simulink model "dsp_blr_hikaku_nakamura_futagi"  (R2018a)
settings: Solver=VariableStepAuto  StartTime=0.0  StopTime=100e-6  RelTol=1e-3
values from neighbouring files (symbols this model uses):
  BASELINE = 0    [dsp_blr.mat]
libraries: xbsIndex_r4 x934, xrbsSSR_Library x35, simulink x3, dspsigattribs x2, hdlsllib x2
(part 1 of 6)
settings Model: Creator=1905p  LastModifiedBy=1905p

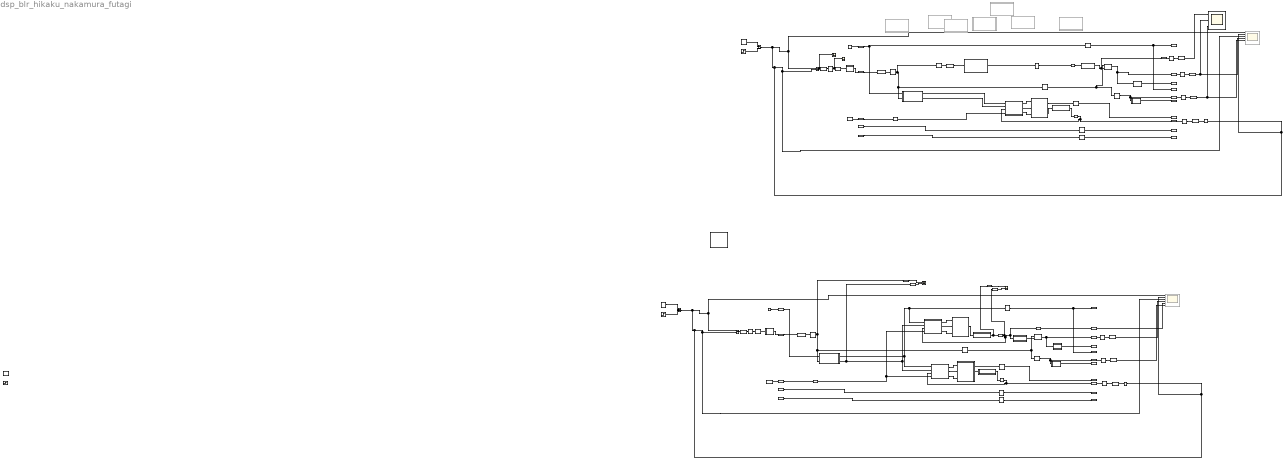
== system dsp_blr_hikaku_nakamura_futagi ==
  note: ここのタイミングはbsp_blr_x.slxのほうで直す
  note: [a:b]を8個用意したが、[0:15]1個ではダメ?
      | 中身は全部同じだった
  note: [a:b]とShiftで入力のvectorと同じ大きさになるようにした
  note: これを入れいるとなぜか上手くいく
  note: 128bitを16bit×8に分け、
      | 足し合わせる
  note: 16×8=128bit
      | のスカラー
  note: 16bit
      | ...
      | 16bit
      | ↑
      | 8行のベクトル
  note: DAC controller
  note: digital_baseline_correction
  note: DSP_module
  note: DAC controller
  note: DSP_module
  note: 16×8=128bit
      | のスカラー
  note: 16bit
      | ...
      | 16bit
      | ↑
      | 8行のベクトル
  note: ここのタイミングはbsp_blr_x.slxのほうで直す
  " System Generator" : xbsIndex_r4/ System Generator  Tag=genX  xilinxfamily=zynquplusRFSOC  part=xczu29dr  speed=-1-e  package=ffvf1760  synthesis_tool=Vivado  clock_wrapper=Clock Enables  directory=C:/Users/1905p/git_repos/KRD/ip_repos/SysGen_outputs/dsp_blr  proj_type=Vivado  Synth_file=Vivado Synthesis Defaults  Impl_file=Vivado Implementation Defaults  testbench=on  simulink_period=8e-9  sysclk_period=8  dcm_input_clock_period=10  incr_netlist=off  trim_vbits=Everywhere in SubSystem  dbl_ovrd=According to Block Masks  core_generation=According to Block Masks  run_coregen=off  deprecated_control=off  eval_field=0  block_type=sysgen
  +cut : Subsystem
  8sample_average 1 : Subsystem
  8sample_average 3 : Subsystem
  "?1" : xbsIndex_r4/Convert  gui_display_data_type=Fixed-point  arith_type="Signed  (2's comp)"  n_bits=16  bin_pt=4  float_type=Single  exp_bits=8  fraction_bits=24  quantization=Truncate  overflow=Saturate  en=off  latency=1  pipeline=off  dbl_ovrd=off  block_type=convert
  Ave10 : Subsystem  Commented=on
  Ave11 : Subsystem
  Ave12 : Subsystem  Commented=on
  Ave5 : Subsystem  Commented=on
  Ave6 : Subsystem  Commented=on
  Ave7 : Subsystem  Commented=on
  Ave8 : Subsystem  Commented=on
  Ave9 : Subsystem  Commented=on
  Buffer1 : Buffer  N=8  OutputFrames=off
  Buffer6 : Buffer  N=8  OutputFrames=off
  Convert 2-D to 1-D1 : dspsigattribs/Convert 2-D to 1-D
      settings: SourceProductName=DSP System Toolbox  SourceProductBaseCode=DS
  Convert 2-D to 1-D6 : dspsigattribs/Convert 2-D to 1-D
      settings: SourceProductName=DSP System Toolbox  SourceProductBaseCode=DS
  Convert1 : xbsIndex_r4/Convert  gui_display_data_type=Fixed-point  arith_type="Signed  (2's comp)"  n_bits=16  bin_pt=4  float_type=Single  exp_bits=8  fraction_bits=24  quantization=Truncate  overflow=Wrap  en=off  latency=0  pipeline=off  dbl_ovrd=off  block_type=convert
  Convert2 : xbsIndex_r4/Convert  gui_display_data_type=Fixed-point  arith_type="Signed  (2's comp)"  n_bits=16  bin_pt=4  float_type=Single  exp_bits=8  fraction_bits=24  quantization=Truncate  overflow=Wrap  en=off  latency=0  pipeline=off  dbl_ovrd=off  block_type=convert
  DAC_M_AXIS_TDATA1 : xbsIndex_r4/Gateway Out  inherit_from_input=on  hdl_port=on  rows=1  columns=1  UseAsDAC=off  DACChannel='1'  interface=None  automatic_assignment=on  address_offset=hex2dec('00')  intf_name=''  intf_description=''  timing_constraint=None  locs_specified=off  LOCs={}  io_standard={}  block_type=gatewayout
  DAC_M_AXIS_TDATA2 : xbsIndex_r4/Gateway Out  inherit_from_input=on  hdl_port=on  rows=1  columns=1  UseAsDAC=off  DACChannel='1'  interface=None  automatic_assignment=on  address_offset=hex2dec('00')  intf_name=''  intf_description=''  timing_constraint=None  locs_specified=off  LOCs={}  io_standard={}  block_type=gatewayout
  DAC_M_AXIS_TVALID1 : xbsIndex_r4/Gateway Out  inherit_from_input=off  hdl_port=on  rows=1  columns=1  UseAsDAC=off  DACChannel='1'  interface=None  automatic_assignment=on  address_offset=hex2dec('00')  intf_name=''  intf_description=''  timing_constraint=None  locs_specified=off  LOCs={}  io_standard={}  block_type=gatewayout
  DAC_M_AXIS_TVALID2 : xbsIndex_r4/Gateway Out  inherit_from_input=off  hdl_port=on  rows=1  columns=1  UseAsDAC=off  DACChannel='1'  interface=None  automatic_assignment=on  address_offset=hex2dec('00')  intf_name=''  intf_description=''  timing_constraint=None  locs_specified=off  LOCs={}  io_standard={}  block_type=gatewayout
  DBL_Scalar2Vector1 : Subsystem
  DBL_Scalar2Vector2 : Subsystem
  DIGITAL_BASELINE4 : xbsIndex_r4/Gateway Out  inherit_from_input=on  hdl_port=on  rows=1  columns=1  UseAsDAC=off  DACChannel='1'  interface=None  automatic_assignment=on  address_offset=hex2dec('00')  intf_name=''  intf_description=''  timing_constraint=None  locs_specified=off  LOCs={}  io_standard={}  block_type=gatewayout
  DSP_M_AXIS_TDATA1 : xbsIndex_r4/Gateway Out  inherit_from_input=on  hdl_port=on  rows=1  columns=1  UseAsDAC=off  DACChannel='1'  interface=None  automatic_assignment=on  address_offset=hex2dec('00')  intf_name=''  intf_description=''  timing_constraint=None  locs_specified=off  LOCs={}  io_standard={}  block_type=gatewayout
  DSP_M_AXIS_TDATA6 : xbsIndex_r4/Gateway Out  inherit_from_input=on  hdl_port=on  rows=1  columns=1  UseAsDAC=off  DACChannel='1'  interface=None  automatic_assignment=on  address_offset=hex2dec('00')  intf_name=''  intf_description=''  timing_constraint=None  locs_specified=off  LOCs={}  io_standard={}  block_type=gatewayout
  DSP_M_AXIS_TDATA_debug1 : xrbsSSR_Library/Vector Real Gateway Out  inherit_from_input=on  hdl_port=off  rows=1  columns=1  UseAsDAC=off  DACChannel='1'  interface=None  automatic_assignment=on  address_offset=hex2dec('00')  intf_name=''  intf_description=''  timing_constraint=None  locs_specified=off  LOCs={}  io_standard={}  block_type=realgatewayout_ssr  sg_ssr=8  sg_ssr_prev=8  sg_ssr_name=vect_real_gwayout
      settings: SourceProductName=Xilinx SSR Blockset  infoedit=The Vector Real Gateway out block converts Xilinx fixed-point or floating-point type vector inputs into vector ouputs of type Simulink integer, single, double, or fixed-point.<br><br>Hardware notes: In hardware these blocks become top level output ports or are discarded, depending on how they are configured.
  DSP_M_AXIS_TDATA_debug2 : xrbsSSR_Library/Vector Real Gateway Out  inherit_from_input=on  hdl_port=off  rows=1  columns=1  UseAsDAC=off  DACChannel='1'  interface=None  automatic_assignment=on  address_offset=hex2dec('00')  intf_name=''  intf_description=''  timing_constraint=None  locs_specified=off  LOCs={}  io_standard={}  block_type=realgatewayout_ssr  sg_ssr=8  sg_ssr_prev=8  sg_ssr_name=vect_real_gwayout
      settings: SourceProductName=Xilinx SSR Blockset  infoedit=The Vector Real Gateway out block converts Xilinx fixed-point or floating-point type vector inputs into vector ouputs of type Simulink integer, single, double, or fixed-point.<br><br>Hardware notes: In hardware these blocks become top level output ports or are discarded, depending on how they are configured.
  DSP_M_AXIS_TDATA_debug7 : xrbsSSR_Library/Vector Real Gateway Out  inherit_from_input=on  hdl_port=off  rows=1  columns=1  UseAsDAC=off  DACChannel='1'  interface=None  automatic_assignment=on  address_offset=hex2dec('00')  intf_name=''  intf_description=''  timing_constraint=None  locs_specified=off  LOCs={}  io_standard={}  block_type=realgatewayout_ssr  sg_ssr=8  sg_ssr_prev=8  sg_ssr_name=vect_real_gwayout
      settings: SourceProductName=Xilinx SSR Blockset  infoedit=The Vector Real Gateway out block converts Xilinx fixed-point or floating-point type vector inputs into vector ouputs of type Simulink integer, single, double, or fixed-point.<br><br>Hardware notes: In hardware these blocks become top level output ports or are discarded, depending on how they are configured.
  DSP_M_AXIS_TVALID1 : xbsIndex_r4/Gateway Out  inherit_from_input=on  hdl_port=on  rows=1  columns=1  UseAsDAC=off  DACChannel='1'  interface=None  automatic_assignment=on  address_offset=hex2dec('00')  intf_name=''  intf_description=''  timing_constraint=None  locs_specified=off  LOCs={}  io_standard={}  block_type=gatewayout
  DSP_M_AXIS_TVALID6 : xbsIndex_r4/Gateway Out  inherit_from_input=on  hdl_port=on  rows=1  columns=1  UseAsDAC=off  DACChannel='1'  interface=None  automatic_assignment=on  address_offset=hex2dec('00')  intf_name=''  intf_description=''  timing_constraint=None  locs_specified=off  LOCs={}  io_standard={}  block_type=gatewayout
  DSP_Vector2Scalar1 : Subsystem
  DSP_Vector2Scalar6 : Subsystem
  DSP_delay1 : xrbsSSR_Library/Vector Delay  sg_latency=7  infoeditControl=Selection of Reset will increase slice count due to use of real FFs and instead of SRLs  en=off  vectorize_en=off  rst=off  reg_retiming=off  block_type=delay_ssr  dbl_ovrd=off  sg_ssr=8  sg_ssr_prev=8  sg_ssr_name=vect_delay
      settings: SourceProductName=Xilinx SSR Blockset
  DSP_delay6 : xrbsSSR_Library/Vector Delay  sg_latency=6  infoeditControl=Selection of Reset will increase slice count due to use of real FFs and instead of SRLs  en=off  vectorize_en=off  rst=off  reg_retiming=off  block_type=delay_ssr  dbl_ovrd=off  sg_ssr=8  sg_ssr_prev=8  sg_ssr_name=vect_delay
      settings: SourceProductName=Xilinx SSR Blockset
  Delay1 : xbsIndex_r4/Delay  rst=off  infoeditControl=Selection of Reset will increase slice count due to use of real FFs and instead of SRLs  en=off  latency=6  reg_retiming=off  dbl_ovrd=off  block_type=delay
  Delay6 : xbsIndex_r4/Delay  rst=off  infoeditControl=Selection of Reset will increase slice count due to use of real FFs and instead of SRLs  en=off  latency=6  reg_retiming=off  dbl_ovrd=off  block_type=delay
  Gateway Out2 : xbsIndex_r4/Gateway Out  inherit_from_input=off  hdl_port=on  rows=1  columns=1  UseAsDAC=off  DACChannel='1'  interface=None  automatic_assignment=on  address_offset=hex2dec('00')  intf_name=''  intf_description=''  timing_constraint=None  locs_specified=off  LOCs={}  io_standard={}  block_type=gatewayout
  Gateway Out3 : xbsIndex_r4/Gateway Out  inherit_from_input=off  hdl_port=on  rows=1  columns=1  UseAsDAC=off  DACChannel='1'  interface=None  automatic_assignment=on  address_offset=hex2dec('00')  intf_name=''  intf_description=''  timing_constraint=None  locs_specified=off  LOCs={}  io_standard={}  block_type=gatewayout
  Gateway Out6 : xbsIndex_r4/Gateway Out  inherit_from_input=off  hdl_port=on  rows=1  columns=1  UseAsDAC=off  DACChannel='1'  interface=None  automatic_assignment=on  address_offset=hex2dec('00')  intf_name=''  intf_description=''  timing_constraint=None  locs_specified=off  LOCs={}  io_standard={}  block_type=gatewayout
  HGAIN_Vector2Scalar1 : Subsystem
  HGAIN_Vector2Scalar6 : Subsystem
  HGAIN_delay1 : xrbsSSR_Library/Vector Delay  sg_latency=1  infoeditControl=Selection of Reset will increase slice count due to use of real FFs and instead of SRLs  en=off  vectorize_en=off  rst=off  reg_retiming=off  block_type=delay_ssr  dbl_ovrd=off  sg_ssr=8  sg_ssr_prev=8  sg_ssr_name=vect_delay
      settings: SourceProductName=Xilinx SSR Blockset
  HGAIN_delay6 : xrbsSSR_Library/Vector Delay  sg_latency=1  infoeditControl=Selection of Reset will increase slice count due to use of real FFs and instead of SRLs  en=off  vectorize_en=off  rst=off  reg_retiming=off  block_type=delay_ssr  dbl_ovrd=off  sg_ssr=8  sg_ssr_prev=8  sg_ssr_name=vect_delay
      settings: SourceProductName=Xilinx SSR Blockset
  H_GAIN_BASELINE1 : xbsIndex_r4/Gateway In  gui_display_data_type=Fixed-point  arith_type="Signed  (2's comp)"  n_bits=13  bin_pt=0  preci_type=Single  exp_width=8  frac_width=24  rows=1  columns=1  quantization=Truncate  overflow=Wrap  period=8e-9  UseAsADC=off  ADCChannel='1'  interface=None  automatic_assignment=on  address_offset=hex2dec('00')  intf_name=''  intf_description=''  default_value=0  timing_constraint=None  locs_specified=off  LOCs={}  io_standard={}  inherit_from_input=off  hdl_port=on  dbl_ovrd=off  block_type=gatewayin
  H_GAIN_BASELINE2 : xbsIndex_r4/Gateway In  gui_display_data_type=Fixed-point  arith_type="Signed  (2's comp)"  n_bits=13  bin_pt=0  preci_type=Single  exp_width=8  frac_width=24  rows=1  columns=1  quantization=Truncate  overflow=Wrap  period=8e-9  UseAsADC=off  ADCChannel='1'  interface=None  automatic_assignment=on  address_offset=hex2dec('00')  intf_name=''  intf_description=''  default_value=0  timing_constraint=None  locs_specified=off  LOCs={}  io_standard={}  inherit_from_input=off  hdl_port=on  dbl_ovrd=off  block_type=gatewayin
  H_M_AXIS_TDATA1 : xbsIndex_r4/Gateway Out  inherit_from_input=on  hdl_port=on  rows=1  columns=1  UseAsDAC=off  DACChannel='1'  interface=None  automatic_assignment=on  address_offset=hex2dec('00')  intf_name=''  intf_description=''  timing_constraint=None  locs_specified=off  LOCs={}  io_standard={}  block_type=gatewayout
  H_M_AXIS_TDATA6 : xbsIndex_r4/Gateway Out  inherit_from_input=on  hdl_port=on  rows=1  columns=1  UseAsDAC=off  DACChannel='1'  interface=None  automatic_assignment=on  address_offset=hex2dec('00')  intf_name=''  intf_description=''  timing_constraint=None  locs_specified=off  LOCs={}  io_standard={}  block_type=gatewayout
  H_M_AXIS_TDATA_debug1 : xrbsSSR_Library/Vector Real Gateway Out  inherit_from_input=on  hdl_port=off  rows=1  columns=1  UseAsDAC=off  DACChannel='1'  interface=None  automatic_assignment=on  address_offset=hex2dec('00')  intf_name=''  intf_description=''  timing_constraint=None  locs_specified=off  LOCs={}  io_standard={}  block_type=realgatewayout_ssr  sg_ssr=8  sg_ssr_prev=8  sg_ssr_name=vect_real_gwayout
      settings: SourceProductName=Xilinx SSR Blockset  infoedit=The Vector Real Gateway out block converts Xilinx fixed-point or floating-point type vector inputs into vector ouputs of type Simulink integer, single, double, or fixed-point.<br><br>Hardware notes: In hardware these blocks become top level output ports or are discarded, depending on how they are configured.
  H_M_AXIS_TDATA_debug6 : xrbsSSR_Library/Vector Real Gateway Out  inherit_from_input=on  hdl_port=off  rows=1  columns=1  UseAsDAC=off  DACChannel='1'  interface=None  automatic_assignment=on  address_offset=hex2dec('00')  intf_name=''  intf_description=''  timing_constraint=None  locs_specified=off  LOCs={}  io_standard={}  block_type=realgatewayout_ssr  sg_ssr=8  sg_ssr_prev=8  sg_ssr_name=vect_real_gwayout
      settings: SourceProductName=Xilinx SSR Blockset  infoedit=The Vector Real Gateway out block converts Xilinx fixed-point or floating-point type vector inputs into vector ouputs of type Simulink integer, single, double, or fixed-point.<br><br>Hardware notes: In hardware these blocks become top level output ports or are discarded, depending on how they are configured.
  H_M_AXIS_TVALID1 : xbsIndex_r4/Gateway Out  inherit_from_input=on  hdl_port=on  rows=1  columns=1  UseAsDAC=off  DACChannel='1'  interface=None  automatic_assignment=on  address_offset=hex2dec('00')  intf_name=''  intf_description=''  timing_constraint=None  locs_specified=off  LOCs={}  io_standard={}  block_type=gatewayout
  H_M_AXIS_TVALID6 : xbsIndex_r4/Gateway Out  inherit_from_input=on  hdl_port=on  rows=1  columns=1  UseAsDAC=off  DACChannel='1'  interface=None  automatic_assignment=on  address_offset=hex2dec('00')  intf_name=''  intf_description=''  timing_constraint=None  locs_specified=off  LOCs={}  io_standard={}  block_type=gatewayout
  H_S_AXIS_TDATA1 : xbsIndex_r4/Gateway In  gui_display_data_type=Fixed-point  arith_type=Unsigned  n_bits=128  bin_pt=0  preci_type=Single  exp_width=8  frac_width=24  rows=1  columns=1  quantization=Truncate  overflow=Wrap  period=8e-9  UseAsADC=off  ADCChannel='1'  interface=None  automatic_assignment=on  address_offset=hex2dec('00')  intf_name=''  intf_description=''  default_value=0  timing_constraint=None  locs_specified=off  LOCs={}  io_standard={}  inherit_from_input=off  hdl_port=on  dbl_ovrd=off  block_type=gatewayin
  H_S_AXIS_TDATA6 : xbsIndex_r4/Gateway In  gui_display_data_type=Fixed-point  arith_type=Unsigned  n_bits=128  bin_pt=0  preci_type=Single  exp_width=8  frac_width=24  rows=1  columns=1  quantization=Truncate  overflow=Wrap  period=8e-9  UseAsADC=off  ADCChannel='1'  interface=None  automatic_assignment=on  address_offset=hex2dec('00')  intf_name=''  intf_description=''  default_value=0  timing_constraint=None  locs_specified=off  LOCs={}  io_standard={}  inherit_from_input=off  hdl_port=on  dbl_ovrd=off  block_type=gatewayin
  H_S_AXIS_TVALID1 : xbsIndex_r4/Gateway In  gui_display_data_type=Boolean  arith_type=Boolean  n_bits=16  bin_pt=14  preci_type=Single  exp_width=8  frac_width=24  rows=1  columns=1  quantization="Round  (unbiased: +/- Inf)"  overflow=Saturate  period=8e-9  UseAsADC=off  ADCChannel='1'  interface=None  automatic_assignment=on  address_offset=hex2dec('00')  intf_name=''  intf_description=''  default_value=0  timing_constraint=None  locs_specified=off  LOCs={}  io_standard={}  inherit_from_input=off  hdl_port=on  dbl_ovrd=off  block_type=gatewayin
  H_S_AXIS_TVALID6 : xbsIndex_r4/Gateway In  gui_display_data_type=Boolean  arith_type=Boolean  n_bits=16  bin_pt=14  preci_type=Single  exp_width=8  frac_width=24  rows=1  columns=1  quantization="Round  (unbiased: +/- Inf)"  overflow=Saturate  period=8e-9  UseAsADC=off  ADCChannel='1'  interface=None  automatic_assignment=on  address_offset=hex2dec('00')  intf_name=''  intf_description=''  default_value=0  timing_constraint=None  locs_specified=off  LOCs={}  io_standard={}  inherit_from_input=off  hdl_port=on  dbl_ovrd=off  block_type=gatewayin
  L_GAIN_TDATA_delay1 : xbsIndex_r4/Delay  rst=off  infoeditControl=Selection of Reset will increase slice count due to use of real FFs and instead of SRLs  en=off  latency=6  reg_retiming=off  dbl_ovrd=off  block_type=delay
  L_GAIN_TDATA_delay6 : xbsIndex_r4/Delay  rst=off  infoeditControl=Selection of Reset will increase slice count due to use of real FFs and instead of SRLs  en=off  latency=6  reg_retiming=off  dbl_ovrd=off  block_type=delay
  L_GAIN_TVALID_delay1 : xbsIndex_r4/Delay  rst=off  infoeditControl=Selection of Reset will increase slice count due to use of real FFs and instead of SRLs  en=off  latency=6  reg_retiming=off  dbl_ovrd=off  block_type=delay
  L_GAIN_TVALID_delay6 : xbsIndex_r4/Delay  rst=off  infoeditControl=Selection of Reset will increase slice count due to use of real FFs and instead of SRLs  en=off  latency=6  reg_retiming=off  dbl_ovrd=off  block_type=delay
  L_M_AXIS_TDATA1 : xbsIndex_r4/Gateway Out  inherit_from_input=on  hdl_port=on  rows=1  columns=1  UseAsDAC=off  DACChannel='1'  interface=None  automatic_assignment=on  address_offset=hex2dec('00')  intf_name=''  intf_description=''  timing_constraint=None  locs_specified=off  LOCs={}  io_standard={}  block_type=gatewayout
  L_M_AXIS_TDATA6 : xbsIndex_r4/Gateway Out  inherit_from_input=on  hdl_port=on  rows=1  columns=1  UseAsDAC=off  DACChannel='1'  interface=None  automatic_assignment=on  address_offset=hex2dec('00')  intf_name=''  intf_description=''  timing_constraint=None  locs_specified=off  LOCs={}  io_standard={}  block_type=gatewayout
  L_M_AXIS_TVALID1 : xbsIndex_r4/Gateway Out  inherit_from_input=on  hdl_port=on  rows=1  columns=1  UseAsDAC=off  DACChannel='1'  interface=None  automatic_assignment=on  address_offset=hex2dec('00')  intf_name=''  intf_description=''  timing_constraint=None  locs_specified=off  LOCs={}  io_standard={}  block_type=gatewayout
  L_M_AXIS_TVALID6 : xbsIndex_r4/Gateway Out  inherit_from_input=on  hdl_port=on  rows=1  columns=1  UseAsDAC=off  DACChannel='1'  interface=None  automatic_assignment=on  address_offset=hex2dec('00')  intf_name=''  intf_description=''  timing_constraint=None  locs_specified=off  LOCs={}  io_standard={}  block_type=gatewayout
  L_S_AXIS_TDATA1 : xbsIndex_r4/Gateway In  gui_display_data_type=Fixed-point  arith_type=Unsigned  n_bits=32  bin_pt=0  preci_type=Single  exp_width=8  frac_width=24  rows=1  columns=1  quantization=Truncate  overflow=Wrap  period=8e-9  UseAsADC=off  ADCChannel='1'  interface=None  automatic_assignment=on  address_offset=hex2dec('00')  intf_name=''  intf_description=''  default_value=0  timing_constraint=None  locs_specified=off  LOCs={}  io_standard={}  inherit_from_input=off  hdl_port=on  dbl_ovrd=off  block_type=gatewayin
  L_S_AXIS_TDATA6 : xbsIndex_r4/Gateway In  gui_display_data_type=Fixed-point  arith_type=Unsigned  n_bits=32  bin_pt=0  preci_type=Single  exp_width=8  frac_width=24  rows=1  columns=1  quantization=Truncate  overflow=Wrap  period=8e-9  UseAsADC=off  ADCChannel='1'  interface=None  automatic_assignment=on  address_offset=hex2dec('00')  intf_name=''  intf_description=''  default_value=0  timing_constraint=None  locs_specified=off  LOCs={}  io_standard={}  inherit_from_input=off  hdl_port=on  dbl_ovrd=off  block_type=gatewayin
  L_S_AXIS_TVALID1 : xbsIndex_r4/Gateway In  gui_display_data_type=Boolean  arith_type=Boolean  n_bits=16  bin_pt=14  preci_type=Single  exp_width=8  frac_width=24  rows=1  columns=1  quantization="Round  (unbiased: +/- Inf)"  overflow=Saturate  period=8e-9  UseAsADC=off  ADCChannel='1'  interface=None  automatic_assignment=on  address_offset=hex2dec('00')  intf_name=''  intf_description=''  default_value=0  timing_constraint=None  locs_specified=off  LOCs={}  io_standard={}  inherit_from_input=off  hdl_port=on  dbl_ovrd=off  block_type=gatewayin
  L_S_AXIS_TVALID6 : xbsIndex_r4/Gateway In  gui_display_data_type=Boolean  arith_type=Boolean  n_bits=16  bin_pt=14  preci_type=Single  exp_width=8  frac_width=24  rows=1  columns=1  quantization="Round  (unbiased: +/- Inf)"  overflow=Saturate  period=8e-9  UseAsADC=off  ADCChannel='1'  interface=None  automatic_assignment=on  address_offset=hex2dec('00')  intf_name=''  intf_description=''  default_value=0  timing_constraint=None  locs_specified=off  LOCs={}  io_standard={}  inherit_from_input=off  hdl_port=on  dbl_ovrd=off  block_type=gatewayin
  Output data Type Conversion DSP1 : DataTypeConversion  OutDataTypeStr=double
  Output data Type Conversion DSP2 : DataTypeConversion  OutDataTypeStr=double
  Output data Type Conversion DSP7 : DataTypeConversion  OutDataTypeStr=double
  Output data Type Conversion HGAIN1 : DataTypeConversion  OutDataTypeStr=double
  Output data Type Conversion HGAIN6 : DataTypeConversion  OutDataTypeStr=double
  Output data Type Conversion1 : DataTypeConversion  OutDataTypeStr=double
  Output data Type Conversion2 : DataTypeConversion  OutDataTypeStr=double
  Scalar2Vector1 : xrbsSSR_Library/Scalar2Vector  Width=16  sg_ssr=8  sg_ssr_prev=8  sg_ssr_name=vect_Scalar2Vector  block_type=scalar2vector_ssr
      settings: SourceProductName=Xilinx SSR Blockset
  Scalar2Vector6 : xrbsSSR_Library/Scalar2Vector  Width=16  sg_ssr=8  sg_ssr_prev=8  sg_ssr_name=vect_Scalar2Vector  block_type=scalar2vector_ssr
      settings: SourceProductName=Xilinx SSR Blockset
  Scope : Scope  NumInputPorts=3
  Scope4 : Scope  NumInputPorts=2
  Scope6 : Scope
  Scope7 : Scope
  Scope8 : Scope  NumInputPorts=2
  Scope_xil1 : Scope  Commented=on  NumInputPorts=6
  Scope_xil2 : Scope  Commented=on  NumInputPorts=6
  Src Switch1 : ManualSwitch
  Src Switch2 : ManualSwitch  CurrentSetting=0
  Src data Type Conversion1 : DataTypeConversion  OutMin=-2048  OutMax=2047  OutDataTypeStr=fixdt(1,16,4)
  Src data Type Conversion6 : DataTypeConversion  OutMin=-2048  OutMax=2047  OutDataTypeStr=fixdt(1,16,4)
  Step1 : Step  Time=50e-6  After=-1024  SampleTime=1e-9
  Step2 : Step  Time=50e-6  After=-1024  SampleTime=1e-9
  Step3 : Step  Time=50e-6  After=-1024  SampleTime=1e-9
  Sum : Sum  Inputs=|+-
  Sum1 : Sum  Inputs=|+-
  Unbuffer DSP1 : Unbuffer
  Unbuffer DSP2 : Unbuffer
  Unbuffer DSP7 : Unbuffer
  Unbuffer HGAIN1 : Unbuffer
  Unbuffer HGAIN6 : Unbuffer
  Unbuffer1 : Unbuffer
  Unbuffer2 : Unbuffer
  Vector AddSub Fabric1 : xrbsSSR_Library/Vector AddSub Fabric  mode=Subtraction  use_carryin=off  use_carryout=off  en=off  sg_latency=1  precision=User Defined  arith_type="Signed  (2's comp)"  n_bits=16  bin_pt=0  quantization=Truncate  overflow=Wrap  use_behavioral_HDL=off  hw_selection=Fabric  pipelined=off  dbl_ovrd=off  block_type=addsub_ssr  sg_ssr=8  sg_ssr_prev=8  sg_ssr_name=vect_addsubfab
      settings: SourceProductName=Xilinx SSR Blockset
  Vector AddSub Fabric2 : xrbsSSR_Library/Vector AddSub Fabric  mode=Subtraction  use_carryin=off  use_carryout=off  en=off  sg_latency=1  precision=User Defined  arith_type="Signed  (2's comp)"  n_bits=16  bin_pt=0  quantization=Truncate  overflow=Wrap  use_behavioral_HDL=off  hw_selection=Fabric  pipelined=off  dbl_ovrd=off  block_type=addsub_ssr  sg_ssr=8  sg_ssr_prev=8  sg_ssr_name=vect_addsubfab
      settings: SourceProductName=Xilinx SSR Blockset
  Vector Real Gateway Out1 : xrbsSSR_Library/Vector Real Gateway Out  inherit_from_input=off  hdl_port=on  rows=1  columns=1  UseAsDAC=off  DACChannel='1'  interface=None  automatic_assignment=on  address_offset=hex2dec('00')  intf_name=''  intf_description=''  timing_constraint=None  locs_specified=off  LOCs={}  io_standard={}  block_type=realgatewayout_ssr  sg_ssr=8  sg_ssr_prev=8  sg_ssr_name=vect_real_gwayout
      settings: SourceProductName=Xilinx SSR Blockset  infoedit=The Vector Real Gateway out block converts Xilinx fixed-point or floating-point type vector inputs into vector ouputs of type Simulink integer, single, double, or fixed-point.<br><br>Hardware notes: In hardware these blocks become top level output ports or are discarded, depending on how they are configured.
  Vector Reinterpret : xrbsSSR_Library/Vector Reinterpret  sg_ssr=8  sg_ssr_prev=8  force_arith_type=on  arith_type=Unsigned  force_bin_pt=on  bin_pt=0  block_type=reinterpret_ssr
      settings: SourceProductName=Xilinx SSR Blockset  infoedit="The Vector Reinterpret block Changes vector input signal type without altering the binary representation. You can change the signal between signed and unsigned, and relocate the binary point.<br><br>Hardware notes: In hardware this block costs nothing.<br><br>Example:  Suppose the input is 6 bits wide, signed, with 2 fractional bits, and the output is forced to unsigned with 0 fractional bits.  Then an input of -2.0 (1110.00 in binary 2's complement) becomes an output of 56 (111000 in binary)."
  Vector Reinterpret1 : xrbsSSR_Library/Vector Reinterpret  sg_ssr=8  sg_ssr_prev=8  force_arith_type=on  arith_type="Signed  (2's comp)"  force_bin_pt=on  bin_pt=4  block_type=reinterpret_ssr
      settings: SourceProductName=Xilinx SSR Blockset  infoedit="The Vector Reinterpret block Changes vector input signal type without altering the binary representation. You can change the signal between signed and unsigned, and relocate the binary point.<br><br>Hardware notes: In hardware this block costs nothing.<br><br>Example:  Suppose the input is 6 bits wide, signed, with 2 fractional bits, and the output is forced to unsigned with 0 fractional bits.  Then an input of -2.0 (1110.00 in binary 2's complement) becomes an output of 56 (111000 in binary)."
  Vector Reinterpret6 : xrbsSSR_Library/Vector Reinterpret  sg_ssr=8  sg_ssr_prev=8  force_arith_type=on  arith_type="Signed  (2's comp)"  force_bin_pt=on  bin_pt=4  block_type=reinterpret_ssr
      settings: SourceProductName=Xilinx SSR Blockset  infoedit="The Vector Reinterpret block Changes vector input signal type without altering the binary representation. You can change the signal between signed and unsigned, and relocate the binary point.<br><br>Hardware notes: In hardware this block costs nothing.<br><br>Example:  Suppose the input is 6 bits wide, signed, with 2 fractional bits, and the output is forced to unsigned with 0 fractional bits.  Then an input of -2.0 (1110.00 in binary 2's complement) becomes an output of 56 (111000 in binary)."
  Vector2Bus1 : Subsystem
  Vector2Bus6 : Subsystem
  Vector2Scalar : xrbsSSR_Library/Vector2Scalar  sg_ssr=8  sg_ssr_prev=8  sg_ssr_name=vect_Vector2Scalar  block_type=vector2scalar_ssr
      settings: SourceProductName=Xilinx SSR Blockset
  Waveform Generator1 : simulink/Sources/Waveform Generator  OutMin=[]  OutMax=[]  OutDataTypeStr=double  SelectedSignal=1  Signals=sin('Amplitude',1024,'Frequency',1000e3,'Phase',0)+square('Amplitude',400,'Frequency',20e6,'Phase',0,'DutyCycle',20)#pulse('Amplitude',1024,'TriggerTime',50e-9,'Duration',50e-9)+step('StepTime',100e-9,'InitialValue',0,'FinalValue',-512)  BlockNames=MultiportSwitch_2ee4ca9575f04b1#MultiportSwitch_74e4ddee714d4bc  SampleTime=1e-9
      settings: SourceProductName=Simulink
  Waveform Generator2 : simulink/Sources/Waveform Generator  OutMin=[]  OutMax=[]  OutDataTypeStr=double  SelectedSignal=1  Signals=sin('Amplitude',1024,'Frequency',1000e3,'Phase',0)+square('Amplitude',400,'Frequency',20e6,'Phase',0,'DutyCycle',20)#pulse('Amplitude',1024,'TriggerTime',50e-9,'Duration',50e-9)+step('StepTime',100e-9,'InitialValue',0,'FinalValue',-512)  BlockNames=MultiportSwitch_2ee4ca9575f04b1#MultiportSwitch_74e4ddee714d4bc  SampleTime=1e-9
      settings: SourceProductName=Simulink
  Waveform Generator3 : simulink/Sources/Waveform Generator  OutMin=[]  OutMax=[]  OutDataTypeStr=double  SelectedSignal=1  Signals=sin('Amplitude',1024,'Frequency',1000e3,'Phase',0)+square('Amplitude',400,'Frequency',20e6,'Phase',0,'DutyCycle',20)#pulse('Amplitude',1024,'TriggerTime',50e-9,'Duration',50e-9)+step('StepTime',100e-9,'InitialValue',0,'FinalValue',-512)  BlockNames=MultiportSwitch_2ee4ca9575f04b1#MultiportSwitch_74e4ddee714d4bc  SampleTime=1e-9
      settings: SourceProductName=Simulink
  baseline1 : Constant  Value=BASELINE  VectorParams1D=off  OutDataTypeStr=Inherit: Inherit via back propagation  SampleTime=1/125e6
  baseline2 : Constant  Value=BASELINE  VectorParams1D=off  OutDataTypeStr=Inherit: Inherit via back propagation  SampleTime=1/125e6
  blr_switch1 : ManualSwitch  CurrentSetting=0
  blr_switch2 : ManualSwitch  CurrentSetting=0
  cast_DBL_out : xbsIndex_r4/Convert  gui_display_data_type=Fixed-point  arith_type="Signed  (2's comp)"  n_bits=16  bin_pt=0  float_type=Single  exp_bits=8  fraction_bits=24  quantization=Truncate  overflow=Wrap  en=off  latency=1  pipeline=off  dbl_ovrd=off  block_type=convert
  convert_to_dac_data2 : xbsIndex_r4/Convert  gui_display_data_type=Fixed-point  arith_type="Signed  (2's comp)"  n_bits=16  bin_pt=4  float_type=Single  exp_bits=8  fraction_bits=24  quantization=Truncate  overflow=Saturate  en=off  latency=1  pipeline=off  dbl_ovrd=off  block_type=convert
  convert_to_dac_input1 : xbsIndex_r4/Convert  gui_display_data_type=Fixed-point  arith_type="Signed  (2's comp)"  n_bits=16  bin_pt=2  float_type=Single  exp_bits=8  fraction_bits=24  quantization=Truncate  overflow=Saturate  en=off  latency=1  pipeline=off  dbl_ovrd=off  block_type=convert
  convert_to_dac_input2 : xbsIndex_r4/Convert  gui_display_data_type=Fixed-point  arith_type="Signed  (2's comp)"  n_bits=16  bin_pt=2  float_type=Single  exp_bits=8  fraction_bits=24  quantization=Truncate  overflow=Saturate  en=off  latency=1  pipeline=off  dbl_ovrd=off  block_type=convert
  ext_delay1 : Delay  DelayLength=3  InitialCondition=0
  ext_delay2 : Delay  DelayLength=3  InitialCondition=0
  tvalid1 : Constant  VectorParams1D=off  OutDataTypeStr=Inherit: Inherit via back propagation  SampleTime=1/125e6
  tvalid6 : Constant  VectorParams1D=off  OutDataTypeStr=Inherit: Inherit via back propagation  SampleTime=1/125e6
  valid_delay1 : xbsIndex_r4/Delay  rst=off  infoeditControl=Selection of Reset will increase slice count due to use of real FFs and instead of SRLs  en=off  latency=1  reg_retiming=off  dbl_ovrd=off  block_type=delay
  valid_delay2 : xbsIndex_r4/Delay  rst=off  infoeditControl=Selection of Reset will increase slice count due to use of real FFs and instead of SRLs  en=off  latency=1  reg_retiming=off  dbl_ovrd=off  block_type=delay
  xil_dac_PID1 : Subsystem
  xil_dac_PID2 : Subsystem
  xil_dac_delta_calc1 : Subsystem
  xil_dac_delta_calc2 : Subsystem
  xil_dac_smoothing1 : Subsystem
  xil_dac_smoothing2 : Subsystem
  xil_dblc_PID1 : Subsystem
  xil_dblc_delta_calc1 : Subsystem
  xil_dblc_smoothing1 : Subsystem
  wires:
  xil_dac_delta_calc1/1(valid_out) -> xil_dac_PID1/1(valid_in)
  ext_delay1/1 -> Scope_xil2/2, Sum/2  "dac_out"
  xil_dac_delta_calc1/2(delta_data_out) -> xil_dac_PID1/2(data_in)
  HGAIN_Vector2Scalar6/1(Out1) -> H_M_AXIS_TDATA6/1
  DSP_M_AXIS_TDATA_debug7/1 -> Unbuffer DSP7/1
  baseline1/1 -> H_GAIN_BASELINE1/1
  L_GAIN_TDATA_delay6/1 -> L_M_AXIS_TDATA6/1
  L_S_AXIS_TDATA6/1 -> L_GAIN_TDATA_delay6/1
  Output data Type Conversion HGAIN6/1 -> Scope_xil2/6  "bypassed_data"
  Unbuffer1/1 -> Output data Type Conversion1/1
  HGAIN_delay6/1 -> H_M_AXIS_TDATA_debug6/1, HGAIN_Vector2Scalar6/1(In1)
  Unbuffer DSP7/1 -> Output data Type Conversion DSP7/1
  8sample_average 3/1(ave_valid_out) -> xil_dac_delta_calc1/1(valid_in), xil_dblc_delta_calc1/1(valid_in), Delay6/1
  Delay6/1 -> DSP_M_AXIS_TVALID6/1, H_M_AXIS_TVALID6/1
  Sum/1 -> blr_switch2/2, Scope_xil2/3  "corrected_out"
  xil_dblc_delta_calc1/1(valid_out) -> xil_dblc_PID1/1(valid_in)
  Output data Type Conversion1/1 -> ext_delay1/1
  blr_switch2/1 -> Src data Type Conversion6/1
  Vector2Bus6/1(Out1) -> H_S_AXIS_TDATA6/1
  Src data Type Conversion6/1 -> Buffer6/1
  Step1/1 -> Src Switch1/2
  xil_dblc_delta_calc1/3(init_pid) -> xil_dblc_PID1/3(init_in)
  valid_delay1/1 -> DAC_M_AXIS_TVALID1/1
  Waveform Generator1/1 -> Src Switch1/1
  Scalar2Vector6/1 -> Vector Reinterpret6/1
  Buffer6/1 -> Convert 2-D to 1-D6/1
  Src Switch1/1 -> blr_switch2/1, Scope_xil2/1, Sum/1  "src_sig"
  tvalid6/1 -> H_S_AXIS_TVALID6/1
  Unbuffer HGAIN6/1 -> Output data Type Conversion HGAIN6/1
  Convert1/1 -> xil_dblc_delta_calc1/4(baseline_in), xil_dac_delta_calc1/4(baseline_in)
  xil_dac_delta_calc1/3(init_pid) -> xil_dac_PID1/3(init_in)
  xil_dac_PID1/1(valid_out) -> valid_delay1/1
  H_GAIN_BASELINE1/1 -> Convert1/1
  DSP_delay6/1 -> HGAIN_delay6/1, Vector AddSub Fabric1/1
  xil_dac_PID1/2(pid_data_out) -> xil_dac_smoothing1/1(data_in)
  convert_to_dac_input1/1 -> DAC_M_AXIS_TDATA1/1, xil_dac_delta_calc1/3(dac_data_in)
  H_S_AXIS_TDATA6/1 -> Scalar2Vector6/1
  cast_DBL_out/1 -> DIGITAL_BASELINE4/1
  DSP_Vector2Scalar6/1(Out1) -> DSP_M_AXIS_TDATA6/1
  xil_dblc_PID1/1(pid_data_out) -> xil_dblc_smoothing1/1(data_in)
  Vector AddSub Fabric1/1 -> DSP_M_AXIS_TDATA_debug7/1, DSP_Vector2Scalar6/1(In1)
  Output data Type Conversion DSP7/1 -> Scope_xil2/4  "dsp_data"
  xil_dblc_delta_calc1/2(delta_data_out) -> xil_dblc_PID1/2(data_in)  "dblc_input"
  L_S_AXIS_TVALID6/1 -> L_GAIN_TVALID_delay6/1
  xil_dac_smoothing1/1(data_out) -> convert_to_dac_input1/1
  H_S_AXIS_TVALID6/1 -> 8sample_average 3/1(valid_in)
  L_GAIN_TVALID_delay6/1 -> L_M_AXIS_TVALID6/1
  H_M_AXIS_TDATA_debug6/1 -> Unbuffer HGAIN6/1
  Convert 2-D to 1-D6/1 -> Vector2Bus6/1(In1)
  Vector Reinterpret6/1 -> Vector Real Gateway Out1/1, 8sample_average 3/2(data_in), DSP_delay6/1
  DIGITAL_BASELINE4/1 -> Scope_xil2/5
  DAC_M_AXIS_TDATA1/1 -> Unbuffer1/1
  L_GAIN_TVALID_delay1/1 -> L_M_AXIS_TVALID1/1
  blr_switch1/1 -> Scope6/1, Src data Type Conversion1/1
  DSP_Vector2Scalar1/1(Out1) -> DSP_M_AXIS_TDATA1/1
  Step3/1 -> Src Switch2/2
  H_S_AXIS_TVALID1/1 -> Delay1/1, 8sample_average 1/1(valid_in)
  Waveform Generator3/1 -> Src Switch2/1
  DSP_delay1/1 -> Vector AddSub Fabric2/1, HGAIN_delay1/1
  L_S_AXIS_TVALID1/1 -> L_GAIN_TVALID_delay1/1
  xil_dac_delta_calc2/3(init_pid) -> xil_dac_PID2/3(init_in)
  H_M_AXIS_TDATA_debug1/1 -> Unbuffer HGAIN1/1
  Buffer1/1 -> Scope7/1, Convert 2-D to 1-D1/1
  H_GAIN_BASELINE2/1 -> Convert2/1
  xil_dac_PID2/2(pid_data_out) -> xil_dac_smoothing2/1(data_in)
  Delay1/1 -> DSP_M_AXIS_TVALID1/1, H_M_AXIS_TVALID1/1
  valid_delay2/1 -> DAC_M_AXIS_TVALID2/1
  tvalid1/1 -> H_S_AXIS_TVALID1/1
  Convert2/1 -> xil_dac_delta_calc2/4(baseline_in)
  Src data Type Conversion1/1 -> Buffer1/1
  Scalar2Vector1/1 -> Vector Reinterpret1/1
  Output data Type Conversion2/1 -> ext_delay2/1
  Src Switch2/1 -> blr_switch1/1, Scope_xil1/1, Sum1/1  "src_sig"
  Sum1/1 -> blr_switch1/2, Scope_xil1/3  "corrected_out"
  8sample_average 1/1(ave_valid_out) -> xil_dac_delta_calc2/1(valid_in)
  L_S_AXIS_TDATA1/1 -> L_GAIN_TDATA_delay1/1
  HGAIN_delay1/1 -> H_M_AXIS_TDATA_debug1/1, HGAIN_Vector2Scalar1/1(In1)
  Output data Type Conversion DSP1/1 -> Scope_xil1/4, Scope/2  "dsp_data"
  DAC_M_AXIS_TDATA2/1 -> Unbuffer2/1
  8sample_average 1/2(ave_data_out) -> xil_dac_delta_calc2/2(data_in)
  Vector Reinterpret1/1 -> Vector Reinterpret/1, 8sample_average 1/2(data_in), DSP_delay1/1
  L_GAIN_TDATA_delay1/1 -> L_M_AXIS_TDATA1/1
  Output data Type Conversion HGAIN1/1 -> Scope_xil1/5, Scope/3  "data"
  Unbuffer2/1 -> Output data Type Conversion2/1
  xil_dac_smoothing2/1(data_out) -> convert_to_dac_input2/1
  convert_to_dac_input2/1 -> DAC_M_AXIS_TDATA2/1, xil_dac_delta_calc2/3(dac_data_in)
  HGAIN_Vector2Scalar1/1(Out1) -> H_M_AXIS_TDATA1/1
  Convert 2-D to 1-D1/1 -> Vector2Bus1/1(In1)
  Unbuffer DSP1/1 -> Output data Type Conversion DSP1/1
  xil_dac_delta_calc2/2(delta_data_out) -> xil_dac_PID2/2(data_in)
  H_S_AXIS_TDATA1/1 -> Scalar2Vector1/1
  Unbuffer HGAIN1/1 -> Output data Type Conversion HGAIN1/1
  baseline2/1 -> H_GAIN_BASELINE2/1
  xil_dac_PID2/1(valid_out) -> valid_delay2/1
  Vector2Bus1/1(Out1) -> H_S_AXIS_TDATA1/1
  xil_dac_delta_calc2/1(valid_out) -> xil_dac_PID2/1(valid_in)
  DSP_M_AXIS_TDATA_debug1/1 -> Unbuffer DSP1/1
  ext_delay2/1 -> Scope_xil1/2, Sum1/2  "dac_out"
  Vector Reinterpret/1 -> Vector2Scalar/1
  Vector2Scalar/1 -> Ave11/1(tdata_in)
  convert_to_dac_data2/1 -> Gateway Out3/1, xil_dblc_delta_calc1/3(blc_data_in), DBL_Scalar2Vector2/1(In1), cast_DBL_out/1
  DBL_Scalar2Vector2/1(Out1) -> Vector AddSub Fabric1/2
  xil_dblc_smoothing1/1(data_out) -> Gateway Out2/1, convert_to_dac_data2/1
  Gateway Out2/1 -> Scope4/1  "before"
  Gateway Out3/1 -> Scope4/2  "after"
  Vector Real Gateway Out1/1 -> Scope8/1  "vector"
  Gateway Out6/1 -> Scope8/2  "scalar"
  8sample_average 3/2(ave_data_out) -> Gateway Out6/1, xil_dac_delta_calc1/2(data_in), xil_dblc_delta_calc1/2(data_in)
  Vector AddSub Fabric2/1 -> DSP_Vector2Scalar1/1(In1), DSP_M_AXIS_TDATA_debug1/1
  "?1"/1 -> DBL_Scalar2Vector1/1(In1)
  Ave11/1(sum_data_out) -> +cut/1(In1)
  +cut/1(Out1) -> "?1"/1
  DBL_Scalar2Vector1/1(Out1) -> DSP_M_AXIS_TDATA_debug2/1, Vector AddSub Fabric2/2
  DSP_M_AXIS_TDATA_debug2/1 -> Unbuffer DSP2/1
  Unbuffer DSP2/1 -> Output data Type Conversion DSP2/1
  Output data Type Conversion DSP2/1 -> Scope/1  "Ave"
